simulink model "ansiOct"  (R2018a)
settings: Solver=VariableStepAuto  StartTime=0.0  StopTime=0.1  RelTol=1e-3
undefined symbols (not defined in the file or in its folder): fdesignblkfcn, G1, G2, G3, G4, G5, G6, G7, G8, gcbh, get, T
libraries: dspsrcs4 x1, dspxfrm3 x1, dspobslib x1
(part 3 of 4)

== system ansiOct/Filter Bank /Filter 3/Bandpass Filter ==
  In : Inport
  Generated Filter Block : DiscreteFir  Tag=BlockMethodSubSystem  Coefficients=[0.000737724855567226264 -7.12621892387676527e-06 -7.10562199524401881e-06 -7.16452421808979412e-06 -7.19265580841319323e-06 -7.29714819573407221e-06 -7.3647135625338432e-06 -7.50199069266997175e-06 -7.59245959456994677e-06 -7.74526175817579297e-06 -7.83946792756576156e-06 -7.98691821420385704e-06 -8.06050340438970738e-06 -8.17689272316811357e-06 -8.20211017609812566e-06 -8.25959963603597479e-06 -8.20608290496499828e-06 -8.17398265284048556e-06 -8.00845283479223867e-06 -7.8545570832792494e-06 -7.54207045642418706e-06 -7.23321829848275345e-06 -6.73706269056869985e-06 -6.24100051915067861e-06 -5.52449943395857804e-06 -4.81198844173254177e-06 -3.83617054920228799e-06 -2.88316809609527731e-06 -1.6049241877129805e-06 -4.09839492108632696e-07 1.23348064266237935e-06 2.5096839854356749e-06 5.85345943053711836e-06 6.75352444634597798e-06 8.50045347500822731e-06 1.09974488099074123e-05 1.34274583614531091e-05 1.62452358983367781e-05 1.91084145381511004e-05 2.2278319148795393e-05 2.55424364923313138e-05 2.90730828715132551e-05 3.27215466823027259e-05 3.66082832980650191e-05 4.06240827770925901e-05 4.48534438170625812e-05 4.92136858445970686e-05 5.37615601348019945e-05 5.84350397020717274e-05 6.326807638338229e-05 6.82157704178995572e-05 7.32910801468407294e-05 7.84650599408803724e-05 8.37304191725084978e-05 8.90747110960299408e-05 9.44682944278114135e-05 9.99177730524242788e-05 0.000105367400983551684 0.000110850507804133416 0.000116275102453098028 0.000121715825188425548 0.000127017048459633191 0.000132342313721611787 0.000137349300933542099 0.000142748449535856018 0.000147469837271089164 0.000151914411212732982 0.000156474080824514704 0.000160652584022318766 0.000164692531547984151 0.000168348340274254027 0.000171767285392595485 0.000174772392745180575 0.00017746607238458041 0.000179705937477423817 0.000181568551703154116 0.000182934843193037169 0.000183863892189233718 0.000184253412596255148 0.000184149257055517648 0.00018346361049363728 0.000182232358596502047 0.000180380865518796503 0.000177936155424388134 0.000174836563462550155 0.000171101187070549535 0.000166682197508253595 0.000161589759505335998 0.000155791375142949297 0.000149286656585544039 0.000142063461766049279 0.000134105896330268638 0.000125429908089196322 0.000115988918033080112 0.000105852877697268897 9.48826361285076209e-05 8.33751498456075006e-05 7.10247895629066223e-05 5.7773325046967753e-05 4.40248800250518646e-05 2.94817620236154808e-05 1.43398367663435126e-05 -1.53870350544853263e-06 -1.80060499347512396e-05 -3.51533536228519213e-05 -5.28535139679296552e-05 -7.11725974459318135e-05 -8.99937421114480756e-05 -0.000109364460702603825 -0.00012917356440912754 -0.000149454561941054001 -0.000170100284127684665 -0.000191132004064357221 -0.000212444880008371106 -0.00023404914491737642 -0.000255842371711342094 -0.000277824655161635747 -0.000299895917105717541 -0.000322046175372417203 -0.000344179029791073104 -0.000366274683874381044 -0.00038824199118040934 -0.000410048954738810568 -0.000431612684758269293 -0.000452886026936947139 -0.000473803950428626117 -0.00049429155076657059 -0.000514332542229477946 -0.000533760738531657798 -0.00055255840775985071 -0.000570856551748353939 -0.000588271854694012307 -0.000604951722990938441 -0.000620710648588873484 -0.000635602532540485753 -0.000649472299078015288 -0.000662350969064199897 -0.000674100685375014406 -0.000684744437222526564 -0.000694156871114877199 -0.00070235718547587958 -0.000709230443783086489 -0.000714795643656427476 -0.000718948363882072439 -0.000721709064631758236 -0.000722983099195099468 -0.000722793426477892392 -0.00072105577273247855 -0.000717796752263790685 -0.000712942640979015245 -0.000706523933314333287 -0.000698478400847819553 -0.000688841201851213844 -0.000677562559155216529 -0.000664680875349856143 -0.000650159702705462375 -0.000634039629869027573 -0.000616302758011205774 -0.000596986569951404628 -0.000576103779162519237 -0.000553673006667855798 -0.000529656886333344052 -0.000504303948047245742 ...(+27601 chars)]  InputProcessing=Columns as channels (frame based)
  Out : Outport
  wires:
  In/1 -> Generated Filter Block/1
  Generated Filter Block/1 -> Out/1

== system ansiOct/Filter Bank /Filter 4/Bandpass Filter ==
  In : Inport
  Generated Filter Block : DiscreteFir  Tag=BlockMethodSubSystem  Coefficients=[0.000769307225021903995 1.39462560566843514e-05 2.24699972520970952e-05 3.64068500121139758e-05 5.53086331206828399e-05 7.86808190633413737e-05 0.000105795968184624811 0.000135942771305882452 0.000168227486094584141 0.00020182536912098138 0.000235765740656352523 0.000269201946079343718 0.000301149008726167588 0.000330808493940412804 0.00035720820806332018 0.000379666498310512069 0.000398969278108317403 0.000410023862765149716 0.000416404925457235144 0.000416198128495857294 0.000408918818882927481 0.000394029627753086768 0.000371114301696191221 0.00033981416451538105 0.000299860390636862476 0.000251078505107380249 0.000193362517905331234 0.000126728267754655792 5.12328038589200891e-05 -3.29077299282083593e-05 -0.000125475345705041742 -0.000226033059270620471 -0.000333634958698509005 -0.000448874113478341563 -0.000569902021380704017 -0.000696195899727076843 -0.000826736043614063757 -0.000960443086110906877 -0.00109608210894339094 -0.00123231094297518895 -0.0013676706994954625 -0.00150060387396832792 -0.00162948519218635121 -0.00175261183810765148 -0.00186827842728686791 -0.00197471962862506368 -0.00207024968936764123 -0.00215313621623837654 -0.00222150761830098697 -0.00227435973226434605 -0.00230972281852849601 -0.00232640288020618657 -0.00232318327633922791 -0.00229906766697730251 -0.00225323542711025919 -0.00218509019015544412 -0.00209426599487450319 -0.00198064740893103301 -0.00184439364454702767 -0.00168592610578865683 -0.00150597806138795987 -0.00130552924551874351 -0.00108590283726323154 -0.000848636659908167442 -0.000595413382812696838 -0.000328635180519285799 -5.03202366766701981e-05 0.000236941952223251482 0.000530482841077111258 0.000827446985635429196 0.00112487374662700998 0.00141971340356509233 0.00170887369880538993 0.00198925734307981578 0.00225779379439734014 0.00251150108289516011 0.00274748869152015599 0.00296306157940862212 0.00315566840424667903 0.00332304784048654839 0.00346329871761103664 0.00357451260795500856 0.00365552143057057237 0.00370529432347032305 0.00372326070430126959 0.00370923188861243701 0.00366345214028484687 0.00358659221260165546 0.0034797570368648007 0.00334447991458345804 0.00318270241760914164 0.00299677555822484235 0.00278939799794479613 0.00256364664087382118 0.00232284971036748238 0.00207064375407317244 0.00181094690098845823 0.00154761104539158823 0.00128487947078322669 0.00102688941472666535 0.000777821825959494097 0.000541766419369416204 0.000322689345929886543 0.00012435986512329049 -4.97074518825848079e-05 -0.000196313501581755231 -0.000312641534658485132 -0.000396292971826617138 -0.000445375021472598463 -0.000458483260440947435 -0.00043483197300291012 -0.000374191324184420149 -0.000276898545388509993 -0.000144105524710283961 2.26016358478678707e-05 0.000220881124234669347 0.000447802973435337186 0.000699812130532160778 0.000972784046388298993 0.00126205637065512194 0.00156248068044047891 0.00186848005442127505 0.00217410516712598315 0.00247312590758029917 0.00275907197811596809 0.00302538289797279472 0.00326540185974130703 0.00347256102148083782 0.00364048469724821081 0.00376289593013927337 0.00383401713976638196 0.00384841603139770769 0.00380121835109366746 0.00368814790303585759 0.00350563023627912217 0.00325086240568497409 0.00292188350122600223 0.00251763512973246289 0.00203800163243973362 0.00148386877661856693 0.000857110383553833237 0.000160673062958747006 -0.000601523649383564575 -0.00142450651234280498 -0.00230226893016691756 -0.00322797032835081456 -0.00419374120058957616 -0.0051909456165646975 -0.00621016172974433404 -0.00724131150216236925 -0.00827374253235710864 -0.00929634272880762447 -0.0102976570251648407 -0.0112660114278864652 -0.0121896542969729509 -0.0130568709487084034 -0.0138561654749222701 -0.0145763234949744178 -0.015206660989739447 -0.015737066599948845 -0.0161581314907620552 -0.0164614159571451028 -0.0166393630630118916 -0.0166855696860778169 -0.0165948059837666001 -0.0163631381236902552 -0.0159879868275143375 -0.0154681913103495387 ...(+5339 chars)]  InputProcessing=Columns as channels (frame based)
  Out : Outport
  wires:
  In/1 -> Generated Filter Block/1
  Generated Filter Block/1 -> Out/1

== system ansiOct/Filter Bank /Filter 5/Bandpass Filter ==
  In : Inport
  Generated Filter Block : DiscreteFir  Tag=BlockMethodSubSystem  Coefficients=[0.000627194137713606983 0.000336773289343153396 0.000408165808565076214 0.000474031977476139013 0.000529332791824150932 0.00056935471293881009 0.000589453675706615643 0.000586070682049277792 0.000556319570000433678 0.000498912510109233076 0.000413697229372969003 0.00030250515074914928 0.000168601543193099842 1.73737823807410018e-05 -0.000144717188991615235 -0.000309671934913568353 -0.000469446899109750456 -0.000615272153224100983 -0.000739218003749897022 -0.000833565180943229888 -0.000892907302673671683 -0.000913696484988393495 -0.000895816278113342811 -0.000840686700903094998 -0.000753220369750108218 -0.000640925677470906502 -0.000516187776608936322 -0.000389227780395694808 -0.000275317431838833701 -0.000189059106243963897 -0.000143502968854972184 -0.000152111423259902246 -0.000223927953498524154 -0.000365739817011667104 -0.00057880806958295354 -0.00086009045259317267 -0.0012004997613373823 -0.00158603592609136155 -0.0019970341210696625 -0.00240977027128702398 -0.00279667239530542516 -0.00312862351283238992 -0.0033756942185857548 -0.00350963085221881648 -0.00350495736367172203 -0.00334156904348817353 -0.00300597777166555346 -0.00249295541651793195 -0.00180605442401004959 -0.000958765146752729963 2.57005863557835629e-05 0.00111491660667590708 0.00226893592640516452 0.00344083119183531076 0.00457995154160260182 0.00563451050950190997 0.00655322016242130493 0.00729007117636976901 0.0078054821539903247 0.00807029515922401929 0.00806713403920111989 0.00779248515832184872 0.00725735507997555662 0.00648758175548629079 0.00552294098500535381 0.0044156161775719821 0.00322750348738164942 0.00202719094077549776 0.000886029056303080454 -0.000125957159911409771 -0.000944552827115539774 -0.00151572254542067276 -0.00179928961057377397 -0.00177257501476462006 -0.00143274986972790545 -0.000798464176828144172 9.00794297116924063e-05 0.00117183676266140787 0.00236720812817520264 0.0035816537947790765 0.00471035058480817354 0.0056431651017419494 0.00627167424034719145 0.00649469912726797702 0.00622556752142813721 0.00539779927159515869 0.00397054467389667924 0.0019330616674483876 -0.000692576616296889476 -0.00384985063100415402 -0.00744841370098850344 -0.0113661467141007531 -0.0154533028918966593 -0.0195380312569094217 -0.0234336744819904248 -0.0269468336720296471 -0.0298867064895119473 -0.0320740171417406156 -0.0333508126482965003 -0.0335885837223063241 -0.0326962001011833064 -0.0306257409526495585 -0.0273769593384601551 -0.0229993041225426305 -0.0175918079351173248 -0.0113005601841151774 -0.0043141542209857919 0.00314352588460663695 0.0108215672144753722 0.0184525091175856797 0.0257632780836048077 0.0324867071280903821 0.0383733019162470976 0.0432017069568407797 0.0467888312803531395 0.0489976442139173282 0.0497434803649952628 0.0489976442139173282 0.0467888312803531395 0.0432017069568407797 0.0383733019162470976 0.0324867071280903821 0.0257632780836048077 0.0184525091175856797 0.0108215672144753722 0.00314352588460663695 -0.0043141542209857919 -0.0113005601841151774 -0.0175918079351173248 -0.0229993041225426305 -0.0273769593384601551 -0.0306257409526495585 -0.0326962001011833064 -0.0335885837223063241 -0.0333508126482965003 -0.0320740171417406156 -0.0298867064895119473 -0.0269468336720296471 -0.0234336744819904248 -0.0195380312569094217 -0.0154533028918966593 -0.0113661467141007531 -0.00744841370098850344 -0.00384985063100415402 -0.000692576616296889476 0.0019330616674483876 0.00397054467389667924 0.00539779927159515869 0.00622556752142813721 0.00649469912726797702 0.00627167424034719145 0.0056431651017419494 0.00471035058480817354 0.0035816537947790765 0.00236720812817520264 0.00117183676266140787 9.00794297116924063e-05 -0.000798464176828144172 -0.00143274986972790545 -0.00177257501476462006 -0.00179928961057377397 -0.00151572254542067276 -0.000944552827115539774 -0.000125957159911409771 0.000886029056303080454 0.00202719094077549776 0.00322750348738164942 0.0044156161775719821 0.00552294098500535381 0.00648758175548629079 ...(+1515 chars)]  InputProcessing=Columns as channels (frame based)
  Out : Outport
  wires:
  In/1 -> Generated Filter Block/1
  Generated Filter Block/1 -> Out/1
